simulink model "virotherapie"  (R2021b)
settings: Solver=VariableStepAuto  StartTime=0.0  StopTime=100  RelTol=1e-3
model workspace (MAT data in the model file):
  IniCond = [126.237 0 2]
settings Model: Creator=danbn  LastModifiedBy=danbn

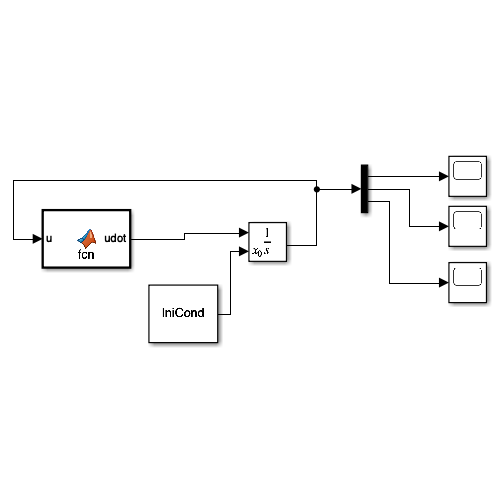
[thumbnail: Simulink's stored preview of the top-level diagram]
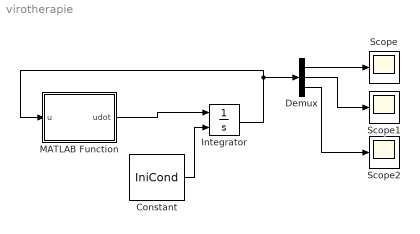
== system virotherapie ==
  Constant : Constant  Value=IniCond
  Demux : Demux  Outputs=3
  Integrator : Integrator  InitialConditionSource=external
  MATLAB Function : MATLAB Function  TreatAsAtomicUnit=on
  Scope : Scope
  Scope1 : Scope
  Scope2 : Scope
  wires:
  MATLAB Function/1(udot) -> Integrator/1
  Integrator/1 -> Demux/1, MATLAB Function/1(u)
  Constant/1 -> Integrator/2
  Demux/1 -> Scope/1
  Demux/2 -> Scope1/1
  Demux/3 -> Scope2/1

== matlab function virotherapie/MATLAB Function ==
  data: u input; udot output
function udot = fcn(u)

r = 0.2062134; %Effective growth rate of uninfected cells day�^-1
K = 2139.258; %Carrying capacity (in 10^6 cells)
kappa = 0.001; %Infection rate constant (per day per 10^6 cells or virions)
rho = 0.2145; %Rate constant of cell fusion (per day per 10^6 cells)
delta = 0.5115; %Effective death rate constant of infected cells day�^-1
omega = 0; %Rate constant of virus elimination day�^-1
alpha = 0; % Virus production rate constant by infected cells (virions per day per cell)
epsilon = 1.64877; %


y = u(1); %Tumor cells 
x = u(2); %Virus infected cell 
v = u(3); %Free virus cells

ydot = r*y*(1-((y+x)/K).^epsilon)-kappa*y*v-rho*x*y;
xdot = kappa*y*v - delta*x;
vdot = alpha*x-omega*v-kappa*y*v;

udot = [ydot,xdot,vdot];
